simulink model "HvCoorn"  (R2022b)
settings: configuration reference "Icar05FusaMdlCfg" (kept outside this file)
undefined symbols (not defined in the file): BMSActSt_ACChrg, BMSActSt_DCChrg, BMSActSt_disconnect, BMSActSt_offline, BMSActSt_online, BMSActSt_undefined, BMSMainNegRlySt_Clsd_SC, BMSMainNegRlySt_Open_SC, BMSMainNegRlySt_StuckInClsd_SC, BMSMainNegRlySt_StuckInOpen_SC, BMSMainPosRlySt_Clsd_SC, BMSMainPosRlySt_Open_SC, BMSMainPosRlySt_StuckInClsd_SC, BMSPrecRlySt_StuckInOpen_SC, BMSReqSt_ACChrg, BMSReqSt_DCChrg, BMSReqSt_emergencyOffline, BMSReqSt_offline, BMSReqSt_online, Chrg_stCycleBookMod_SC, Chrg_stSingleBookMod_SC, CmpgMod_stInactv_SC, DCDCActSt_buck, DCDCActSt_connected, DCDCActSt_disconnected, DCDCReqSt_buck, DCDCReqSt_standby, EngStrtStop_RefuModDft_SC, EPBActSt_Appld_SC, GearLvr_stDrvGearD_SC, GearLvr_stDrvGearN_SC, GearLvr_stDrvGearP_SC, GearLvr_stDrvGearR_SC, hpp_bACChargeLinkIni_C, hpp_bACChargeLinkOKIni_C, hpp_bAcChgEnaIni_C, hpp_bAcChgPauseIni_C, hpp_bAcLinkTempErrIni_C, hpp_bBattWarmReqIni_C, hpp_bHvilHwErrIni_C, hpp_bHvilStOkIni_C, hpp_bHvRelayClsActIni_C, hpp_bHvRelayOpnActIni_C, hpp_bHvRelayStuckIni_C, hpp_bParked4ChDchgIni_C, hpp_bRemLvBatMntnReqIni_C, hpp_bStartUpReqIni_C, hpp_stHvilCanIni_C, hpp_stWarmTimeCfgRespIni_C, HvCoorn_bAuthEnaSwt_C, HvCoorn_bAuthFailSpdLimOvrd_C, HvCoorn_bAuthFailSpdLimOvrdVal_C, HvCoorn_bAuthStrt_C, HvCoorn_bBMSUnexpdDcnctFailEna_C, HvCoorn_bBuck2RdyBypDCDCEna_C, HvCoorn_bDCChrgFctCfg_C, HvCoorn_bDcChrgWkupEnaChrgLink_C, HvCoorn_bDCDcnct4ACEna_C, HvCoorn_bDCNotBuck2ShtdwnEna_C, HvCoorn_bDrvrLevNotRdyEna_C ... (+295)
libraries: ITKLib x213, simulink x61
(part 10 of 12)

== system HvCoorn/HvCoorn/HVP_HighVoltagePowerOnOffProcedure/A01_HighvoltPowerUpReq/B07_AcChrgPwrUp ==
  note: This subsystem calculates AC charge enable flag and AC charge wake up vehicle high voltage power up flag.
  note: Documentation
  HvCoorn_bACLinkTempErr : Inport
  HvCoorn_bParked4ChDchg : Inport  Port=2
  Chrg_bACChrgCmpl : Inport  Port=3
  iud_stOBCWakeUpOrigin : Inport  Port=4
  icobc_bChrgrCtrlSigCnct : Inport  Port=5
  icbms_bBatACChrgFull : Inport  Port=6
  Chrg_stBookChrgMod : Inport  Port=7
  HvCoorn_bObcChrgrCnct : Inport  Port=8
  HvCoorn_bACChrgLink : Inport  Port=9
  icobc_pwrChrgMax : Inport  Port=10
  HvCoorn_bBattWarmReq : Inport  Port=11
  Chrg_bBookChrgCmpl : Inport  Port=12
  HvCoorn_bACChrgLinkOk : Inport  Port=13
  Chrg_bChrgStopBySOCLim : Inport  Port=14
  Chrg_bChrgErrForever : Inport  Port=15
  Constant10 : Constant  Description=[254]  Value=HvCoorn_noACChrgEna_C
      settings: AttributesFormatString=%<Description>
  Copyright : simulink/Model-Wide Utilities/Model Info  Frame=on  DisplayStringWithTags=|  HorizontalTextAlignment=Left  LeftAlignmentValue=0.02
      | © ITK Engineering Technology (Wu Xi) Co., Ltd. (ITKC)
      | 
      | Model Version: %<ModelVersion>
      | Date: %<LastModificationDate>
  InlineDescription : ITKLib/Special/InlineDescription  Tag=HideFromReport  Description=AC充电上高压  ShowInLibBrowser=0  RefreshPar=0
      settings: SourceProductName=ITKC_Lib
  Logical Operator1 : Logic  AllPortsSameDT=off  OutDataTypeStr=boolean
  Logical Operator{2,4..5,10,24} (5 alike) : Logic  Operator=NOT  Inputs=1  AllPortsSameDT=off  OutDataTypeStr=boolean
  Logical Operator17 : Logic  Operator=OR  Inputs=3  AllPortsSameDT=off  OutDataTypeStr=boolean
  Logical Operator18 : Logic  AllPortsSameDT=off  OutDataTypeStr=boolean
  Logical Operator20 : Logic  Operator=OR  Inputs=3  AllPortsSameDT=off  OutDataTypeStr=boolean
  Logical Operator23 : Logic  Operator=OR  AllPortsSameDT=off  OutDataTypeStr=boolean
  Logical Operator31 : Logic  Operator=OR  AllPortsSameDT=off  OutDataTypeStr=boolean
  MaskAnd : ITKLib/BitOperation/MaskAnd
      settings: SourceProductName=ITKC_Lib
  Merge8bit2out : ITKLib/BitOperation/Merge8bit2out
      settings: AttributesFormatString=Merge8bit2out  SourceProductName=ITKC_Lib
  OR : Logic  Operator=OR  Inputs=3  OutDataTypeStr=boolean
  RSLatch : ITKLib/Memory/RSLatch
      settings: SourceProductName=ITKC_Lib
  RSLatch1 : ITKLib/Memory/RSLatch
      settings: SourceProductName=ITKC_Lib
  Relational Operator{3,5..6,10..11} (5 alike) : RelationalOperator  Operator===  OutDataTypeStr=boolean  InputSameDT=off
  Relational Operator7 : RelationalOperator  OutDataTypeStr=boolean  InputSameDT=off
  Unit Delay3 : UnitDelay  SampleTime=-1  HasFrameUpgradeWarning=on
      settings: AttributesFormatString=<initial=%<X0>>
  Unit detailed design : simulink/Model-Wide Utilities/DocBlock  Tag=HideFromReport  DocumentType=Text
      content=|
      | SMiVCU-3258 - AC充电使能
      | 以下条件同时满足，则激活[AC充电使能]：
      | 1.<充电激活输出状态>激活，且<OBC充电连接状态>为0x2：Connected激活并锁存，[AC充电连接标志位]为0时Reset；
      | 2.[AC充电连接OK标志位]为1且<BMS充电使能>为0x1：Enable；
      | 3.[停车运行充放电标志位]为1；
      | 4.<OBC当前可输出最大功率>大于一定值（HvCoorn_pwrOBCSplyLim_C，初始值500V）；
      | 5.<交流充电充满标志位>为0x0：Not full；
      | 6.<充电持续故障>为0；
      |
      | SMiVCU-3259 - AC充电高压请求标志位
      | [AC充电使能]激活且<AC充电完成标志位>为0在，则激活并锁存[AC充电高压请求标志位]，<AC充电完成标志位>为1Reset。
  hpp_bEpbPark4ChDchgEna_C4 : Constant  Description=[3]  Value=Chrg_stCycleBookMod_SC
      settings: AttributesFormatString=%<Description>
  hpp_bEpbPark4ChDchgEna_C5 : Constant  Description=[2]  Value=Chrg_stSingleBookMod_SC
      settings: AttributesFormatString=%<Description>
  hpp_pwrIpsSplyLim_C : Constant  Description=[0]  Value=HvCoorn_pwrOBCSplyLim_C
      settings: AttributesFormatString=%<Description>
  uint1 : Constant  Description=CCWake  Value=96  OutDataTypeStr=uint8
      settings: AttributesFormatString=|
      | %<OutDataTypeStr>
      | %<Description>
  uint2 : Constant  Description=CPWake  Value=97  OutDataTypeStr=uint8
      settings: AttributesFormatString=|
      | %<OutDataTypeStr>
      | %<Description>
  uint8 : Constant  Description=IgWake  Value=18  OutDataTypeStr=uint8
      settings: AttributesFormatString=|
      | %<OutDataTypeStr>
      | %<Description>
  HvCoorn_bACChrgEna : Outport  VectorParamsAs1DForOutWhenUnconnected=off
  HvCoorn_bACChrgPwrUp : Outport  Port=2  VectorParamsAs1DForOutWhenUnconnected=off
  wires:
  Logical Operator10/1 -> Logical Operator1/2
  Logical Operator1/1 -> RSLatch1/1
  iud_stOBCWakeUpOrigin/1 -> Relational Operator5/1, Relational Operator3/1, Relational Operator6/1
  uint2/1 -> Relational Operator6/2
  Relational Operator5/1 -> Logical Operator17/1
  Logical Operator18/1 -> Unit Delay3/1
  Logical Operator17/1 -> Logical Operator20/1  "WakeUpOrigin"
  Unit Delay3/1 -> Logical Operator20/2  "RePlugOrSwipCard"
  icbms_bBatACChrgFull/1 -> Logical Operator24/1
  Logical Operator24/1 -> Logical Operator23/1
  HvCoorn_bBattWarmReq/1 -> Logical Operator23/2
  Relational Operator6/1 -> Logical Operator17/3
  Relational Operator3/1 -> Logical Operator17/2
  uint1/1 -> Relational Operator3/2
  uint8/1 -> Relational Operator5/2
  MaskAnd/1 -> Logical Operator1/1, HvCoorn_bACChrgEna/1
  icobc_bChrgrCtrlSigCnct/1 -> Merge8bit2out/2, Logical Operator18/1
  HvCoorn_bObcChrgrCnct/1 -> Logical Operator18/2
  Chrg_stBookChrgMod/1 -> Relational Operator10/1, Relational Operator11/1
  hpp_bEpbPark4ChDchgEna_C4/1 -> Relational Operator10/2
  hpp_bEpbPark4ChDchgEna_C5/1 -> Relational Operator11/2
  Relational Operator11/1 -> Logical Operator31/2
  Relational Operator10/1 -> Logical Operator31/1
  Logical Operator31/1 -> Logical Operator20/3  "BookChg"
  RSLatch1/1 -> HvCoorn_bACChrgPwrUp/1  "HvCoorn_bACChrgPwrUp"
  Logical Operator20/1 -> RSLatch/1
  HvCoorn_bACChrgLink/1 -> Logical Operator2/1
  Logical Operator2/1 -> RSLatch/2
  RSLatch/1 -> Merge8bit2out/1  "bAcChgTrig"
  HvCoorn_bACLinkTempErr/1 -> Logical Operator5/1
  HvCoorn_bParked4ChDchg/1 -> Merge8bit2out/5
  Logical Operator5/1 -> Merge8bit2out/4
  Logical Operator23/1 -> Merge8bit2out/7
  Relational Operator7/1 -> Merge8bit2out/6
  hpp_pwrIpsSplyLim_C/1 -> Relational Operator7/2
  icobc_pwrChrgMax/1 -> Relational Operator7/1
  Chrg_bChrgErrForever/1 -> Logical Operator4/1
  Logical Operator4/1 -> Merge8bit2out/8
  Merge8bit2out/1 -> MaskAnd/1  "HvCoorn_noACChrgEnaBitVal"
  Constant10/1 -> MaskAnd/2
  HvCoorn_bACChrgLinkOk/1 -> Merge8bit2out/3
  OR/1 -> RSLatch1/2, Logical Operator10/1
  Chrg_bChrgStopBySOCLim/1 -> OR/2
  Chrg_bACChrgCmpl/1 -> OR/1
  Chrg_bBookChrgCmpl/1 -> OR/3

== system HvCoorn/HvCoorn/HVP_HighVoltagePowerOnOffProcedure/A01_HighvoltPowerUpReq/B08_DcChrgPwrUp ==
  note: This subsystem calculates DC charge enable flag and DC charge wake up vehicle high voltage power up flag.
  note: Documentation
  Chrg_bChrgStopBySOCLim : Inport
  Chrg_bChrgErrForever : Inport  Port=2
  HvCoorn_bDcLinkTempErr : Inport  Port=3
  HvCoorn_bParked4ChDchg : Inport  Port=4
  HvCoorn_bDCChrgLink : Inport  Port=5
  icbms_bDcChrgCfg : Inport  Port=6
  Chrg_bDCChrgCmpl : Inport  Port=7
  icbms_bBatDCChrgFull : Inport  Port=8
  icbms_uDcChgrCap : Inport  Port=9
  icbms_iDcChgrCap : Inport  Port=10
  icbms_bDcChrgWkup : Inport  Port=11
  AND : Logic  Inputs=8  OutDataTypeStr=boolean
  AND1 : Logic  OutDataTypeStr=boolean
  Copyright : simulink/Model-Wide Utilities/Model Info  Frame=on  DisplayStringWithTags=|  HorizontalTextAlignment=Left  LeftAlignmentValue=0.02
      | © ITK Engineering Technology (Wu Xi) Co., Ltd. (ITKC)
      | 
      | Model Version: %<ModelVersion>
      | Date: %<LastModificationDate>
  GreaterOrEqual : RelationalOperator  OutDataTypeStr=boolean
  InlineDescription : ITKLib/Special/InlineDescription  Tag=HideFromReport  Description=DC充电上高压  ShowInLibBrowser=0  RefreshPar=0
      settings: SourceProductName=ITKC_Lib
  Logical Operator1 : Logic  Operator=NOT  AllPortsSameDT=off  OutDataTypeStr=boolean
  Logical Operator2 : Logic  Operator=NOT  AllPortsSameDT=off  OutDataTypeStr=boolean
  Logical Operator4 : Logic  Operator=NOT  Inputs=1  AllPortsSameDT=off  OutDataTypeStr=boolean
  Logical Operator9 : Logic  Operator=NOT  AllPortsSameDT=off  OutDataTypeStr=boolean
  OR : Logic  Operator=OR  OutDataTypeStr=boolean
  Product : Product  InputSameDT=on  SaturateOnIntegerOverflow=on
  RSLatch : ITKLib/Memory/RSLatch
      settings: SourceProductName=ITKC_Lib
  Unit detailed design : simulink/Model-Wide Utilities/DocBlock  Tag=HideFromReport  DocumentType=Text
      content=|
      | SMiVCU-3265 - DC充电使能
      | 以下条件同时满足，则激活[DC充电使能]：
      | 1.[DC充电连接标志位]为1;
      | 2.[DC充电充满标志位]为0；
      | 3.[停车运行充放电标志位]为1；
      | 4.<直流充电激活状态>为1；
      | 5.<充电持续故障>为0；
      |
      | SMiVCU-3266 - DC充电高压请求标志位
      | [DC充电使能]激活，且<DC充电完成标志位>为0，则激活并锁存[DC充电高压请求标志位]，<DC充电完成标志位>为1则Reset。
  hpp_pwrIpsSplyLim_C1 : Constant  Description=[0]  Value=HvCoorn_pwrDCChrgrSplyLim_C
      settings: AttributesFormatString=%<Description>
  HvCoorn_bDCChrgEna : Outport  VectorParamsAs1DForOutWhenUnconnected=off
  HvCoorn_bDCChrgPwrUp : Outport  Port=2  VectorParamsAs1DForOutWhenUnconnected=off
  wires:
  AND/1 -> HvCoorn_bDCChrgEna/1, AND1/1
  Logical Operator2/1 -> AND1/2
  AND1/1 -> RSLatch/1
  RSLatch/1 -> HvCoorn_bDCChrgPwrUp/1  "HvCoorn_bDCChrgPwrUp"
  icbms_bBatDCChrgFull/1 -> Logical Operator9/1
  HvCoorn_bDCChrgLink/1 -> AND/1
  icbms_bDcChrgCfg/1 -> AND/2
  Logical Operator9/1 -> AND/3
  HvCoorn_bDcLinkTempErr/1 -> Logical Operator1/1
  Logical Operator1/1 -> AND/4
  HvCoorn_bParked4ChDchg/1 -> AND/5
  icbms_uDcChgrCap/1 -> Product/1
  icbms_iDcChgrCap/1 -> Product/2
  hpp_pwrIpsSplyLim_C1/1 -> GreaterOrEqual/2
  Product/1 -> GreaterOrEqual/1
  GreaterOrEqual/1 -> AND/6
  icbms_bDcChrgWkup/1 -> AND/7
  Chrg_bChrgErrForever/1 -> Logical Operator4/1
  Logical Operator4/1 -> AND/8
  OR/1 -> Logical Operator2/1, RSLatch/2
  Chrg_bDCChrgCmpl/1 -> OR/1
  Chrg_bChrgStopBySOCLim/1 -> OR/2

== system HvCoorn/HvCoorn/HVP_HighVoltagePowerOnOffProcedure/A01_HighvoltPowerUpReq/B09_KeyOnPwrUp ==
  note: Documentation
  idi_bKeyOn : Inport
  icbms_pctHVBatSOCDisp : Inport  Port=2
  PwrLimBatt_pwrMaxHvesDChrg : Inport  Port=3
  idi_bKeyStrt : Inport  Port=4
  HvCoorn_bHvReady : Inport  Port=5
  BrkPedDev_bBrk : Inport  Port=6
  iczcu_bHVPwrOffReq : Inport  Port=7
  HvCoorn_stHVPOld : Inport  Port=8
  icicm_bPwrOffReq : Inport  Port=9
  GearLvr_stDrvGear : Inport  Port=10
  HvCoorn_bChrgLink : Inport  Port=11
  icicm_bOTAOn : Inport  Port=12
  DrvMod_bVehShowMod : Inport  Port=13
  icbms_stHvBat : Inport  Port=14
  AND : Logic  OutDataTypeStr=boolean
  AND1 : Logic  Inputs=3  OutDataTypeStr=boolean
  Copyright : simulink/Model-Wide Utilities/Model Info  Frame=on  DisplayStringWithTags=|  HorizontalTextAlignment=Left  LeftAlignmentValue=0.02
      | © ITK Engineering Technology (Wu Xi) Co., Ltd. (ITKC)
      | 
      | Model Version: %<ModelVersion>
      | Date: %<LastModificationDate>
  EdgeFalling : ITKLib/Memory/EdgeFalling  Tag=initial value = 0
      settings: SourceProductName=ITKC_Lib
  EdgeRising : ITKLib/Memory/EdgeRising  Tag=initial value = 0
      settings: SourceProductName=ITKC_Lib
  EdgeRising1 : ITKLib/Memory/EdgeRising  Tag=initial value = 0
      settings: SourceProductName=ITKC_Lib
  EdgeRising2 : ITKLib/Memory/EdgeRising  Tag=initial value = 0
      settings: SourceProductName=ITKC_Lib
  Equal : RelationalOperator  Operator===  OutDataTypeStr=boolean  RndMeth=Simplest  InputSameDT=off
  Equal1 : RelationalOperator  Operator===  OutDataTypeStr=boolean  RndMeth=Simplest  InputSameDT=off
  HysteresisB : ITKLib/Hysteresis/HysteresisB  Description=HysteresisB
      settings: AttributesFormatString=%<Description>  SourceProductName=ITKC_Lib
  InlineDescription : ITKLib/Special/InlineDescription  Tag=HideFromReport  Description=KeyOn上高压  ShowInLibBrowser=0  RefreshPar=0
      settings: SourceProductName=ITKC_Lib
  Logical Operator{1,3..5,7} (5 alike) : Logic  AllPortsSameDT=off  OutDataTypeStr=boolean
  Logical Operator14 : Logic  Operator=NOT  Inputs=1  AllPortsSameDT=off  OutDataTypeStr=boolean
  Logical Operator15 : Logic  Inputs=3  AllPortsSameDT=off  OutDataTypeStr=boolean
  Logical Operator2 : Logic  Inputs=3  AllPortsSameDT=off  OutDataTypeStr=boolean
  LowerOrEqual : RelationalOperator  Operator=<=  OutDataTypeStr=boolean
  LowerOrEqual1 : RelationalOperator  OutDataTypeStr=boolean
  LowerOrEqual2 : RelationalOperator  Operator===  OutDataTypeStr=boolean
  NOT : Logic  Operator=NOT  AllPortsSameDT=off  OutDataTypeStr=boolean
  NOT1 : Logic  Operator=NOT  AllPortsSameDT=off  OutDataTypeStr=boolean
  Not : Logic  Operator=NOT  AllPortsSameDT=off  OutDataTypeStr=boolean
  Not1 : Logic  Operator=NOT  AllPortsSameDT=off  OutDataTypeStr=boolean
  Not2 : Logic  Operator=NOT  AllPortsSameDT=off  OutDataTypeStr=boolean
  OR{,1..2,4,6..7} (6 alike) : Logic  Operator=OR  OutDataTypeStr=boolean
  OR3 : Logic  OutDataTypeStr=boolean
  OR5 : Logic  Inputs=4  OutDataTypeStr=boolean
  OR8 : Logic  Operator=OR  Inputs=3  OutDataTypeStr=boolean
  RSLatch : ITKLib/Memory/RSLatch
      settings: SourceProductName=ITKC_Lib
  RSLatch1 : ITKLib/Memory/RSLatch
      settings: SourceProductName=ITKC_Lib
  Relational Operator3 : RelationalOperator  Operator=<  OutDataTypeStr=boolean  InputSameDT=off
  Relational Operator4 : RelationalOperator  Operator=<  OutDataTypeStr=boolean  InputSameDT=off
  Relational Operator5 : RelationalOperator  Operator=~=  OutDataTypeStr=boolean  InputSameDT=off
  Relational Operator6 : RelationalOperator  Operator=~=  OutDataTypeStr=boolean  InputSameDT=off
  Switch : Switch  Criteria=u2 ~= 0  SaturateOnIntegerOverflow=off  InputSameDT=off
      settings: AttributesFormatString=Criteria : %<Criteria>
  Switch1 : Switch  Criteria=u2 ~= 0  SaturateOnIntegerOverflow=off  InputSameDT=off
      settings: AttributesFormatString=Criteria : %<Criteria>
  TRUE : Constant  Description=TRUE  OutDataTypeStr=boolean
      settings: AttributesFormatString=%<Description>
  TRUE1 : Constant  Description=TRUE  OutDataTypeStr=boolean  SampleTime=-1
      settings: AttributesFormatString=%<Description>
  TaskTime_s1 : Constant  Value=TaskTime_10ms
      settings: AttributesFormatString=[0.01]
  TaskTime_s2 : Constant  Value=TaskTime_10ms
      settings: AttributesFormatString=[0.01]
  TaskTime_s3 : Constant  Value=TaskTime_10ms
      settings: AttributesFormatString=[0.01]
  TurnOnDelayVari1 : ITKLib/TimeCounter/TurnOnDelayVari
      settings: AttributesFormatString=TurnOnDelay  SourceProductName=ITKC_Lib
  TurnOnDelayVari2 : ITKLib/TimeCounter/TurnOnDelayVari
      settings: AttributesFormatString=TurnOnDelay  SourceProductName=ITKC_Lib
  Turn_Off_Delay_Vari : ITKLib/TimeCounter/Turn_Off_Delay_Vari
      settings: AttributesFormatString=TurnOffDelay  SourceProductName=ITKC_Lib
  Unit detailed design : simulink/Model-Wide Utilities/DocBlock  Tag=HideFromReport  DocumentType=Text
      content=|
      | SMiVCU-3273 - KeyOn高压请求标志位
      | 以下条件同时满足，则激活[KeyOn高压请求标志位]：
      | 1.<整车电源模式>为0x1：On，TurnOnDelay一定时间（HvCoorn_tiKeyOnDly_C，初始值0.05s）出现上升沿，则激活并锁存。
      | 若<高压下电指令>为1 TurnOnDelay一定时间（HvCoorn_tiPwrOffDly4RstKeyOn_C，初始值0.2s），或<整车电源模式>为0x0：off，或当前时刻<高压系统状态>在115~130之间出现上升沿Reset；
      | 2.<电池SOC>大于等于一定值（HvCoorn_pctBatSOCLim4Shut_C，初始值0.01）或<电池最大放电功率>大于等于一定值（hpp_pwrBatDChrgLim4Shut_C，初始值1000W）；
  UnitDelay : UnitDelay  SampleTime=-1  HasFrameUpgradeWarning=on
      settings: AttributesFormatString=<Initial=%<x0>>
  hpp_bEpbPark4ChDchgEna_C2 : Constant  Description=[6]  Value=GearLvr_stDrvGearP_SC  OutDataTypeStr=uint8
      settings: AttributesFormatString=%<Description>
  hpp_bEpbPark4ChDchgEna_C4 : Constant  Description=[4]  Value=GearLvr_stDrvGearN_SC  OutDataTypeStr=uint8
      settings: AttributesFormatString=%<Description>
  hpp_percBatDchgSocThre_C : Constant  Description=[0]  Value=HvCoorn_pctBatSOCLim4Shut_C
      settings: AttributesFormatString=%<Description>
  hpp_percBatDchgSocThre_C1 : Constant  Description=[1]  Value=HvCoorn_bKeyOnStrtHvEna_C
      settings: AttributesFormatString=%<Description>
  hpp_percBatDchgSocThre_C2 : Constant  Description=[1]  Value=HvCoorn_bKeyStrtStrtHvEna_C
      settings: AttributesFormatString=%<Description>
  hpp_percBatDchgSocThre_C3 : Constant  Description=[1]  Value=HvCoorn_bSOPVehKeyOnStrtHvEna_C
      settings: AttributesFormatString=%<Description>
  hpp_percBatDchgSocThre_C4 : Constant  Description=[10]  Value=HvCoorn_tiVehShowLoSocInhbOn_C
      settings: AttributesFormatString=%<Description>
  hpp_percBatDchgSocThre_C5 : Constant  Description=[0.2]  Value=HvCoorn_tiPwrOffDly4RstKeyOn_C
      settings: AttributesFormatString=%<Description>
  hpp_percBatDchgSocThre_C6 : Constant  Description=[0.03]  Value=HvCoorn_tiKeyOnRisKeep_C
      settings: AttributesFormatString=%<Description>
  hpp_percBatDchgSocThre_C7 : Constant  Description=[0]  Value=HvCoorn_bZCUPwrOffEna_C
      settings: AttributesFormatString=%<Description>
  hpp_pwrSocHiBatDchgThre_C : Constant  Description=[-5000]  Value=HvCoorn_pwrBatDChrgLim4Shut_C
      settings: AttributesFormatString=%<Description>
  hpp_pwrSocHiBatDchgThre_C1 : Constant  Description=[1]  Value=HvCoorn_bVehShowLoSocInhbKeyOnEna_C
      settings: AttributesFormatString=%<Description>
  hpp_pwrSocHiBatDchgThre_C2 : Constant  Description=[6]  Value=HvCoorn_pctVehShowLoSocInhbOnUppr_C
      settings: AttributesFormatString=%<Description>
  hpp_pwrSocHiBatDchgThre_C3 : Constant  Description=[4]  Value=HvCoorn_pctVehShowLoSocInhbOnLowr_C
      settings: AttributesFormatString=%<Description>
  icbms_acCharge : Constant  Description=[9]  Value=BMSActSt_ACChrg  OutDataTypeStr=uint8
      settings: AttributesFormatString=[9]
  icbms_dcCharge : Constant  Description=[8]  Value=BMSActSt_DCChrg  OutDataTypeStr=uint8
      settings: AttributesFormatString=[8]
  single : Constant  Value=101  OutDataTypeStr=uint8  SampleTime=-1
      settings: AttributesFormatString=%<OutDataTypeStr>
  single1 : Constant  Value=130  OutDataTypeStr=uint8  SampleTime=-1
      settings: AttributesFormatString=%<OutDataTypeStr>
  single2 : Constant  Value=89  OutDataTypeStr=uint8  SampleTime=-1
      settings: AttributesFormatString=%<OutDataTypeStr>
  sup_tiKeyStrt_C1 : Constant  Description=[0]  Value=HvCoorn_bKeyStrtBypBrkSwt_C
      settings: AttributesFormatString=%<Description>
  HvCoorn_bKeyOnPwrUp : Outport  VectorParamsAs1DForOutWhenUnconnected=off
  HvCoorn_bShowModSocLo : Outport  Port=2  VectorParamsAs1DForOutWhenUnconnected=off
  wires:
  idi_bKeyOn/1 -> Logical Operator1/1, [idi_bKeyOn]
  Logical Operator15/1 -> HvCoorn_bKeyOnPwrUp/1  "HvCoorn_bKeyOnPwrUp"
  PwrLimBatt_pwrMaxHvesDChrg/1 -> Relational Operator4/1
  icbms_pctHVBatSOCDisp/1 -> [icbms_pctHVBatSOCDisp], Relational Operator3/1
  hpp_percBatDchgSocThre_C/1 -> Relational Operator3/2
  hpp_pwrSocHiBatDchgThre_C/1 -> Relational Operator4/2
  Relational Operator4/1 -> Logical Operator7/2
  Relational Operator3/1 -> Logical Operator7/1
  Logical Operator7/1 -> Logical Operator14/1
  Logical Operator14/1 -> Logical Operator15/2
  hpp_percBatDchgSocThre_C1/1 -> Logical Operator1/2
  hpp_percBatDchgSocThre_C2/1 -> Logical Operator2/2
  idi_bKeyStrt/1 -> Logical Operator2/1
  RSLatch/1 -> Switch/3
  Logical Operator3/1 -> Logical Operator15/1
  HvCoorn_bHvReady/1 -> UnitDelay/1
  TRUE/1 -> Switch/1
  Switch/1 -> Logical Operator3/2
  sup_tiKeyStrt_C1/1 -> OR1/2
  BrkPedDev_bBrk/1 -> OR1/1
  OR1/1 -> Logical Operator2/3
  Logical Operator2/1 -> RSLatch/1
  NOT/1 -> RSLatch/2
  OR/1 -> Switch/2
  hpp_percBatDchgSocThre_C3/1 -> OR/1
  UnitDelay/1 -> OR/2
  Turn_Off_Delay_Vari/1 -> RSLatch1/1  "HvCoorn_bKeyOnRisSet"
  iczcu_bHVPwrOffReq/1 -> OR4/1
  TaskTime_s2/1 -> TurnOnDelayVari1/2
  hpp_percBatDchgSocThre_C5/1 -> TurnOnDelayVari1/3
  RSLatch1/1 -> Logical Operator3/1
  OR2/1 -> EdgeRising1/1
  TurnOnDelayVari1/1 -> OR2/1
  EdgeRising1/1 -> OR7/1
  HvCoorn_stHVPOld/1 -> [HvCoorn_stHVPOld], LowerOrEqual/1, LowerOrEqual1/1
  single/1 -> LowerOrEqual1/2
  single1/1 -> LowerOrEqual/2
  LowerOrEqual/1 -> OR3/1
  LowerOrEqual1/1 -> OR3/2
  OR3/1 -> OR2/2
  OR5/1 -> TurnOnDelayVari1/1
  icicm_bPwrOffReq/1 -> OR4/2
  OR4/1 -> OR5/1
  GearLvr_stDrvGear/1 -> Equal/1, Equal1/1
  hpp_bEpbPark4ChDchgEna_C2/1 -> Equal/2
  hpp_bEpbPark4ChDchgEna_C4/1 -> Equal1/2
  Equal/1 -> OR6/1
  Equal1/1 -> OR6/2
  OR6/1 -> OR5/4
  HvCoorn_bChrgLink/1 -> Not/1
  Not/1 -> OR5/3
  NOT1/1 -> OR7/2
  [idi_bKeyOn] -> NOT1/1
  [idi_bKeyOn] -> NOT/1
  TaskTime_s3/1 -> Turn_Off_Delay_Vari/2
  hpp_percBatDchgSocThre_C6/1 -> Turn_Off_Delay_Vari/3
  OR7/1 -> RSLatch1/2
  hpp_percBatDchgSocThre_C7/1 -> OR5/2
  Logical Operator1/1 -> Logical Operator4/1, Logical Operator5/1, EdgeRising/1
  EdgeFalling/1 -> Logical Operator4/2
  icicm_bOTAOn/1 -> EdgeFalling/1
  Logical Operator4/1 -> OR8/2
  EdgeRising/1 -> OR8/3
  Logical Operator5/1 -> OR8/1
  single2/1 -> LowerOrEqual2/2
  LowerOrEqual2/1 -> EdgeRising2/1
  EdgeRising2/1 -> Logical Operator5/2
  [HvCoorn_stHVPOld] -> LowerOrEqual2/1
  OR8/1 -> Turn_Off_Delay_Vari/1
  Switch1/1 -> Not2/1, Logical Operator15/3
  TRUE1/1 -> Switch1/3
  AND/1 -> Switch1/2
  DrvMod_bVehShowMod/1 -> AND/1
  hpp_pwrSocHiBatDchgThre_C1/1 -> AND/2
  [icbms_pctHVBatSOCDisp] -> HysteresisB/2
  hpp_pwrSocHiBatDchgThre_C2/1 -> HysteresisB/1
  icbms_acCharge/1 -> Relational Operator6/2
  icbms_dcCharge/1 -> Relational Operator5/2
  icbms_stHvBat/1 -> Relational Operator5/1, Relational Operator6/1
  Relational Operator5/1 -> AND1/2
  Relational Operator6/1 -> AND1/1
  hpp_percBatDchgSocThre_C4/1 -> TurnOnDelayVari2/3
  TaskTime_s1/1 -> TurnOnDelayVari2/2
  AND1/1 -> TurnOnDelayVari2/1
  Not1/1 -> Switch1/1
  TurnOnDelayVari2/1 -> Not1/1
  Not2/1 -> HvCoorn_bShowModSocLo/1
  HysteresisB/1 -> AND1/3
  hpp_pwrSocHiBatDchgThre_C3/1 -> HysteresisB/3

== system HvCoorn/HvCoorn/HVP_HighVoltagePowerOnOffProcedure/A01_HighvoltPowerUpReq/B10_RemotePwrUp ==
  note: This subsystem calculates Tbox remote wake up vehicle high voltage power up flag.
  ictel_stHvBatPrecdng : Inport
  tcj_bHvBatPrecdngFinish : Inport  Port=2
  iczcu_stRmtChrgReq : Inport  Port=3
  iud_stRemoteImmo : Inport  Port=4
  ipf_bBD1CAN0x41CVld : Inport  Port=5
  ictcp_stRmtHvReq : Inport  Port=6
  idi_bKeyOn : Inport  Port=7
  icbms_pctHVBatSOCDisp : Inport  Port=8
  Equal : RelationalOperator  Operator===  OutDataTypeStr=boolean  RndMeth=Simplest  InputSameDT=off
  Equal1 : RelationalOperator  Operator===  OutDataTypeStr=boolean  RndMeth=Simplest  InputSameDT=off
  Logical Operator1 : Logic  Operator=OR  AllPortsSameDT=off  OutDataTypeStr=boolean
  Logical Operator34 : Logic  Operator=OR  Inputs=3  AllPortsSameDT=off  OutDataTypeStr=boolean
  Logical Operator35 : Logic  AllPortsSameDT=off  OutDataTypeStr=boolean
  Logical Operator36 : Logic  Operator=OR  AllPortsSameDT=off  OutDataTypeStr=boolean
  Logical Operator9 : Logic  Operator=OR  Inputs=3  AllPortsSameDT=off  OutDataTypeStr=boolean
  Not : Logic  Operator=NOT  AllPortsSameDT=off  OutDataTypeStr=boolean
  OR : Logic  Operator=OR  Inputs=3  OutDataTypeStr=boolean
  RSLatch : ITKLib/Memory/RSLatch
      settings: SourceProductName=ITKC_Lib
  RSLatch1 : ITKLib/Memory/RSLatch
      settings: SourceProductName=ITKC_Lib
  RSLatch2 : ITKLib/Memory/RSLatch
      settings: SourceProductName=ITKC_Lib
  Relational Operator10 : RelationalOperator  Operator=<  OutDataTypeStr=boolean  InputSameDT=off
  Relational Operator{3..5,14..17} (7 alike) : RelationalOperator  Operator===  OutDataTypeStr=boolean  InputSameDT=off
  TaskTime_s1 : Constant  Value=TaskTime_10ms
      settings: AttributesFormatString=[0.01]
  TaskTime_s2 : Constant  Value=TaskTime_10ms
      settings: AttributesFormatString=[0.01]
  Terminator : Terminator
  TurnOnDelayVari : ITKLib/TimeCounter/TurnOnDelayVari
      settings: AttributesFormatString=TurnOnDelay  SourceProductName=ITKC_Lib
  TurnOnDelayVari1 : ITKLib/TimeCounter/TurnOnDelayVari
      settings: AttributesFormatString=TurnOnDelay  SourceProductName=ITKC_Lib
  hpp_bReMoteImmoEna_C : Constant  Description=[1]  Value=HvCoorn_bRemImobEna_C  OutDataTypeStr=boolean
      settings: AttributesFormatString=%<Description>
  hpp_tiRemHvBatPrecdngSet_C : Constant  Description=[0.01]  Value=HvCoorn_tiRemHvBatPreCdngSet_C
      settings: AttributesFormatString=%<Description>
  hpp_tiRemLvBatMntnSet_C : Constant  Description=[0.01]  Value=HvCoorn_tiRemLvBatMntnSet_C
      settings: AttributesFormatString=%<Description>
  sup_percSocAdj4HvOn_C : Constant  Description=[15]  Value=HvCoorn_pctSocRmtHvRstThd_C
      settings: AttributesFormatString=%<Description>
  uint1 : Constant  Description=Cycle  Value=2  OutDataTypeStr=uint8
      settings: AttributesFormatString=|
      | %<OutDataTypeStr>
      | %<Description>
  uint2 : Constant  Description=Single  Value=4  OutDataTypeStr=uint8
      settings: AttributesFormatString=|
      | %<OutDataTypeStr>
      | %<Description>
  uint3 : Constant  Description=Start  Value=6  OutDataTypeStr=uint8
      settings: AttributesFormatString=|
      | %<OutDataTypeStr>
      | %<Description>
  uint4 : Constant  Description=HV active  OutDataTypeStr=uint8
      settings: AttributesFormatString=|
      | %<OutDataTypeStr>
      | %<Description>
  uint5 : Constant  Description=HV not active  Value=2  OutDataTypeStr=uint8
      settings: AttributesFormatString=|
      | %<OutDataTypeStr>
      | %<Description>
  uint6 : Constant  Description=Released  Value=2  OutDataTypeStr=uint8
      settings: AttributesFormatString=|
      | %<OutDataTypeStr>
      | %<Description>
  uint7 : Constant  Description=Charge Req  OutDataTypeStr=uint8
      settings: AttributesFormatString=|
      | %<OutDataTypeStr>
      | %<Description>
  uint8 : Constant  Description=Charge Finished  Value=2  OutDataTypeStr=uint8
      settings: AttributesFormatString=|
      | %<OutDataTypeStr>
      | %<Description>
  uint9 : Constant  Description=Charge Req  Value=0  OutDataTypeStr=uint8
      settings: AttributesFormatString=|
      | %<OutDataTypeStr>
      | %<Description>
  HvCoorn_bRemPwrUp : Outport  VectorParamsAs1DForOutWhenUnconnected=off
  wires:
  TaskTime_s2/1 -> TurnOnDelayVari/2
  Logical Operator34/1 -> TurnOnDelayVari/1  "bHvBatPrecdng"
  tcj_bHvBatPrecdngFinish/1 -> RSLatch/2
  iczcu_stRmtChrgReq/1 -> Relational Operator3/1, Relational Operator5/1, Relational Operator4/1
  hpp_tiRemHvBatPrecdngSet_C/1 -> TurnOnDelayVari/3
  TurnOnDelayVari1/1 -> RSLatch1/1
  RSLatch/1 -> Logical Operator1/2
  uint1/1 -> Relational Operator14/2
  uint2/1 -> Relational Operator15/2
  uint3/1 -> Relational Operator16/2
  Relational Operator14/1 -> Logical Operator34/1
  Relational Operator15/1 -> Logical Operator34/2
  Relational Operator16/1 -> Logical Operator34/3
  ictel_stHvBatPrecdng/1 -> Relational Operator15/1, Relational Operator16/1, Relational Operator14/1
  uint6/1 -> Relational Operator17/2
  iud_stRemoteImmo/1 -> Relational Operator17/1
  Logical Operator35/1 -> TurnOnDelayVari1/1
  Logical Operator36/1 -> Logical Operator35/2
  Relational Operator17/1 -> Logical Operator36/1
  hpp_bReMoteImmoEna_C/1 -> Logical Operator36/2
  hpp_tiRemLvBatMntnSet_C/1 -> TurnOnDelayVari1/3
  Logical Operator1/1 -> HvCoorn_bRemPwrUp/1  "HvCoorn_bRemPwrUp"
  TurnOnDelayVari/1 -> RSLatch/1
  TaskTime_s1/1 -> TurnOnDelayVari1/2
  Relational Operator3/1 -> Logical Operator35/1
  uint7/1 -> Relational Operator3/2
  uint8/1 -> Relational Operator4/2
  Logical Operator9/1 -> RSLatch1/2
  uint9/1 -> Relational Operator5/2
  Relational Operator4/1 -> Logical Operator9/1
  Relational Operator5/1 -> Logical Operator9/2
  ipf_bBD1CAN0x41CVld/1 -> Not/1
  Not/1 -> Logical Operator9/3
  ictcp_stRmtHvReq/1 -> Equal1/1, Equal/1
  uint4/1 -> Equal/2
  Equal/1 -> RSLatch2/1
  RSLatch2/1 -> Logical Operator1/1
  Equal1/1 -> OR/1
  uint5/1 -> Equal1/2
  OR/1 -> RSLatch2/2
  idi_bKeyOn/1 -> OR/2
  RSLatch1/1 -> Terminator/1
  icbms_pctHVBatSOCDisp/1 -> Relational Operator10/1
  sup_percSocAdj4HvOn_C/1 -> Relational Operator10/2
  Relational Operator10/1 -> OR/3

== system HvCoorn/HvCoorn/HVP_HighVoltagePowerOnOffProcedure/A01_HighvoltPowerUpReq/B11_ECCPwrUp ==
  note: Documentation
  icecc_bHVReq : Inport
  icems_bFanAftRunActv : Inport  Port=2
  HvCoorn_bKeyOnPwrUp : Inport  Port=3
  AND : Logic  OutDataTypeStr=boolean
  AND1 : Logic  OutDataTypeStr=boolean
  Copyright : simulink/Model-Wide Utilities/Model Info  Frame=on  DisplayStringWithTags=|  HorizontalTextAlignment=Left  LeftAlignmentValue=0.02
      | © ITK Engineering Technology (Wu Xi) Co., Ltd. (ITKC)
      | 
      | Model Version: %<ModelVersion>
      | Date: %<LastModificationDate>
  EdgeFalling : ITKLib/Memory/EdgeFalling  Tag=initial value = 0
      settings: SourceProductName=ITKC_Lib
  InlineDescription : ITKLib/Special/InlineDescription  Tag=HideFromReport  Description=热管理上高压  ShowInLibBrowser=0  RefreshPar=0
      settings: SourceProductName=ITKC_Lib
  NormShut1 : Constant  Description=[1]  Value=HvCoorn_bECCPwrUpEna_C
      settings: AttributesFormatString=%<Description>
  Not : Logic  Operator=NOT  AllPortsSameDT=off  OutDataTypeStr=boolean
  OR : Logic  Operator=OR  OutDataTypeStr=boolean
  OR1 : Logic  Operator=OR  OutDataTypeStr=boolean
  RSLatch : ITKLib/Memory/RSLatch
      settings: SourceProductName=ITKC_Lib
  TaskTime_s1 : Constant  Value=TaskTime_10ms
      settings: AttributesFormatString=[0.01]
  TurnOnDelayVari1 : ITKLib/TimeCounter/TurnOnDelayVari
      settings: AttributesFormatString=TurnOnDelay  SourceProductName=ITKC_Lib
  Unit Delay : UnitDelay  SampleTime=-1  HasFrameUpgradeWarning=on
      settings: AttributesFormatString=<initial=%<x0>>
  Unit detailed design : simulink/Model-Wide Utilities/DocBlock  Tag=HideFromReport  DocumentType=Text
      content=|
      | SMiVCU-3269 - 热管理高压请求标志位
      | 以下条件同时满足，则激活[热管理高压请求标志位]：
      | 1.[热管理高压请求]为1；
      | 2.[热管理可用最大功率]大于一定值（HvCoorn_pwrEccEnaHv_C，初始值1W）。
  hpp_tiRemLvBatMntnSet_C : Constant  Description=[600]  Value=HvCoorn_tiFanAftRunMaxThd_C
      settings: AttributesFormatString=%<Description>
  HvCoorn_bECCPwrUp : Outport
  wires:
  icecc_bHVReq/1 -> AND/1
  NormShut1/1 -> AND/2
  HvCoorn_bKeyOnPwrUp/1 -> EdgeFalling/1
  EdgeFalling/1 -> AND1/1
  icems_bFanAftRunActv/1 -> Not/1, AND1/2
  AND/1 -> OR/1
  OR/1 -> HvCoorn_bECCPwrUp/1
  RSLatch/1 -> OR/2, Unit Delay/1  "HvCoorn_bFanAftRunPwrUp"
  AND1/1 -> RSLatch/1
  Not/1 -> OR1/1
  OR1/1 -> RSLatch/2
  hpp_tiRemLvBatMntnSet_C/1 -> TurnOnDelayVari1/3
  TaskTime_s1/1 -> TurnOnDelayVari1/2
  TurnOnDelayVari1/1 -> OR1/2
  Unit Delay/1 -> TurnOnDelayVari1/1

== system HvCoorn/HvCoorn/HVP_HighVoltagePowerOnOffProcedure/A01_HighvoltPowerUpReq/B12_OTAPwrUp ==
  icicm_bOTAOn : Inport
  icicm_stHVReq : Inport  Port=2
  AND : Logic  OutDataTypeStr=boolean
  AND1 : Logic  OutDataTypeStr=boolean
  Equal : RelationalOperator  Operator===  OutDataTypeStr=boolean  RndMeth=Simplest  InputSameDT=off
  Equal1 : RelationalOperator  Operator===  OutDataTypeStr=boolean  RndMeth=Simplest  InputSameDT=off
  uint1 : Constant  Value=2  OutDataTypeStr=uint8  SampleTime=-1
      settings: AttributesFormatString=%<OutDataTypeStr>
  uint8 : Constant  OutDataTypeStr=uint8  SampleTime=-1
      settings: AttributesFormatString=%<OutDataTypeStr>
  HvCoorn_bOTAPwrUp : Outport
  HvCoorn_bOTAHvOffReq : Outport  Port=2
  wires:
  icicm_stHVReq/1 -> Equal1/1, Equal/1
  uint8/1 -> Equal/2
  Equal/1 -> AND/2
  AND/1 -> HvCoorn_bOTAPwrUp/1
  icicm_bOTAOn/1 -> AND1/1, AND/1
  Equal1/1 -> AND1/2
  uint1/1 -> Equal1/2
  AND1/1 -> HvCoorn_bOTAHvOffReq/1

== system HvCoorn/HvCoorn/HVP_HighVoltagePowerOnOffProcedure/A01_HighvoltPowerUpReq/B13_GatherPwrUpReq ==
  note: This subsystem calculates high voltage start up request flag, based on AC charge, DC charge, Key on, remote power up.
  note: Documentation
  HvCoorn_bACChrgPwrUp : Inport
  HvCoorn_bDCChrgPwrUp : Inport  Port=2
  HvCoorn_bKeyOnPwrUp : Inport  Port=3
  ved_bHvShtdwn : Inport  Port=4
  icbms_bHvShutOffReq : Inport  Port=5
  HvCoorn_bRemPwrUp : Inport  Port=6
  HvCoorn_bECCPwrUp : Inport  Port=7
  HvCoorn_bOTAPwrUp : Inport  Port=8
  HvCoorn_bOTAHvOffReq : Inport  Port=9
  GearLvr_stDrvGear : Inport  Port=10
  icbms_pctHVBatSOCDisp : Inport  Port=11
  iczcu_stCarMod : Inport  Port=12
  HvCoorn_bV2LActv : Inport  Port=13
  ved_bInhbHvOn : Inport  Port=14
  HvCoorn_stHVPOld : Inport  Port=15
  HvCoorn_bHvOnFai : Inport  Port=16
  HvCoorn_bHvInitFail : Inport  Port=17
  HvCoorn_bRemLvBatMntnReq : Inport  Port=18
  RngPrdn_volFuRmnByInstModEEW : Inport  Port=19
  ved_bInhbEngStrt : Inport  Port=20
  ved_bCellVoltUndLimSrus : Inport  Port=21
  AND : Logic  Inputs=4  OutDataTypeStr=boolean
  AND1 : Logic  OutDataTypeStr=boolean
  AND2 : Logic  OutDataTypeStr=boolean
  Calibration6 : Constant  Description=[3]  Value=HvCoorn_volTankRmnFuLowrTranMod_C  SampleTime=-1
      settings: AttributesFormatString=%<Description>
  Copyright : simulink/Model-Wide Utilities/Model Info  Frame=on  DisplayStringWithTags=|  HorizontalTextAlignment=Left  LeftAlignmentValue=0.02
      | © ITK Engineering Technology (Wu Xi) Co., Ltd. (ITKC)
      | 
      | Model Version: %<ModelVersion>
      | Date: %<LastModificationDate>
  Equal1 : RelationalOperator  Operator=<=  OutDataTypeStr=boolean  RndMeth=Simplest  InputSameDT=off
  Equal2 : RelationalOperator  Operator===  OutDataTypeStr=boolean
  Equal3 : RelationalOperator  OutDataTypeStr=boolean  RndMeth=Simplest  InputSameDT=off
  Equal4 : RelationalOperator  Operator=<  OutDataTypeStr=boolean
  Equal5 : RelationalOperator  Operator===  OutDataTypeStr=boolean  RndMeth=Simplest  InputSameDT=off
  Equal6 : RelationalOperator  Operator===  OutDataTypeStr=boolean  RndMeth=Simplest  InputSameDT=off
  InlineDescription : ITKLib/Special/InlineDescription  Tag=HideFromReport  Description=高压上电请求  ShowInLibBrowser=0  RefreshPar=0
      settings: SourceProductName=ITKC_Lib
  Logical Operator{1..5} (5 alike) : Logic  Operator=NOT  Inputs=1  AllPortsSameDT=off  OutDataTypeStr=boolean
  Logical Operator26 : Logic  Inputs=6  AllPortsSameDT=off  OutDataTypeStr=boolean
  Merge8bit2out : ITKLib/BitOperation/Merge8bit2out
      settings: AttributesFormatString=Merge8bit2out  SourceProductName=ITKC_Lib
  Not : Logic  Operator=NOT  AllPortsSameDT=off  OutDataTypeStr=boolean
  OR : Logic  Operator=OR  Inputs=3  OutDataTypeStr=boolean
  OR1 : Logic  Operator=OR  Inputs=6  OutDataTypeStr=boolean
  OR2 : Logic  Operator=OR  OutDataTypeStr=boolean
  OR3 : Logic  Operator=OR  Inputs=3  OutDataTypeStr=boolean
  OR4 : Logic  Operator=OR  OutDataTypeStr=boolean
  OR5 : Logic  Operator=OR  OutDataTypeStr=boolean
  Relational Operator10 : RelationalOperator  Operator=<=  OutDataTypeStr=boolean  InputSameDT=off
  TaskTime_s1 : Constant  Description=[4]  Value=GearLvr_stDrvGearN_SC  SampleTime=-1
      settings: AttributesFormatString=%<Description>
  TaskTime_s2 : Constant  Description=[6]  Value=GearLvr_stDrvGearP_SC  SampleTime=-1
      settings: AttributesFormatString=%<Description>
  TaskTime_s3 : Constant  Value=TaskTime_10ms
      settings: AttributesFormatString=[0.01]
  TurnOnDelayVari : ITKLib/TimeCounter/TurnOnDelayVari
      settings: AttributesFormatString=TurnOnDelay  SourceProductName=ITKC_Lib
  Unit detailed design : simulink/Model-Wide Utilities/DocBlock  Tag=HideFromReport  DocumentType=Text
      content=|
      | SMiVCU-3271 - 上高压需求标志位
      | 以下任一条件满足，且<整车故障等级>小于4，且<BMS高压断开请求>为0，则激活[上高压需求标志位]
      | 1.[AC充电高压请求标志位]为1；
      | 2.[DC充电高压请求标志位]；
      | 3.[KeyOn高压请求标志位]；
      | 4.[热管理高压请求标志位]，且热管理上高压使能标志位（HvCoorn_bECCPwrUpEna_C，初始值0）为1。
  hpp_percBatDchgSocThre_C6 : Constant  Description=[0.3]  Value=HvCoorn_tiCarModPwrOffDly_C
      settings: AttributesFormatString=%<Description>
  sup_percSocAdj4HvOn_C : Constant  Description=[10]  Value=HvCoorn_pctSocTransptHvOff_C
      settings: AttributesFormatString=%<Description>
  uint1 : Constant  Value=2  OutDataTypeStr=uint8  SampleTime=-1
      settings: AttributesFormatString=%<OutDataTypeStr>
  uint2 : Constant  Value=10  OutDataTypeStr=uint8  SampleTime=-1
      settings: AttributesFormatString=%<OutDataTypeStr>
  uint3 : Constant  Value=101  OutDataTypeStr=uint8  SampleTime=-1
      settings: AttributesFormatString=%<OutDataTypeStr>
  HvCoorn_bStartUpReq : Outport  VectorParamsAs1DForOutWhenUnconnected=off
  HvCoorn_stStartUpReq : Outport  Port=2  VectorParamsAs1DForOutWhenUnconnected=off
  wires:
  HvCoorn_bACChrgPwrUp/1 -> OR/1, Merge8bit2out/1
  Logical Operator26/1 -> HvCoorn_bStartUpReq/1
  HvCoorn_bKeyOnPwrUp/1 -> Merge8bit2out/4, OR1/2
  HvCoorn_bRemPwrUp/1 -> OR1/1, Merge8bit2out/3
  HvCoorn_bDCChrgPwrUp/1 -> OR/2, Merge8bit2out/2
  Logical Operator1/1 -> Logical Operator26/2
  icbms_bHvShutOffReq/1 -> Logical Operator1/1
  HvCoorn_bECCPwrUp/1 -> OR1/4, Merge8bit2out/6
  Logical Operator2/1 -> Logical Operator26/3
  HvCoorn_bOTAPwrUp/1 -> Merge8bit2out/5, OR1/3
  HvCoorn_bOTAHvOffReq/1 -> Logical Operator3/1
  Logical Operator3/1 -> Logical Operator26/4
  Merge8bit2out/1 -> HvCoorn_stStartUpReq/1
  HvCoorn_bV2LActv/1 -> OR1/5, Merge8bit2out/7
  GearLvr_stDrvGear/1 -> Equal6/1, Equal5/1
  TaskTime_s2/1 -> Equal5/2
  sup_percSocAdj4HvOn_C/1 -> Relational Operator10/2
  icbms_pctHVBatSOCDisp/1 -> Relational Operator10/1
  uint1/1 -> Equal2/2  "TransportMode"
  iczcu_stCarMod/1 -> Equal2/1
  Relational Operator10/1 -> AND/2
  Equal2/1 -> AND/3
  AND/1 -> Not/1
  OR1/1 -> AND1/1
  AND1/1 -> OR/3
  OR/1 -> Logical Operator26/1
  ved_bHvShtdwn/1 -> Logical Operator2/1
  ved_bInhbHvOn/1 -> OR3/1
  AND2/1 -> Logical Operator4/1
  Logical Operator4/1 -> Logical Operator26/6
  HvCoorn_stHVPOld/1 -> Equal3/1, Equal1/1
  Equal1/1 -> OR2/1
  OR2/1 -> AND2/2
  Equal3/1 -> OR2/2
  uint2/1 -> Equal1/2
  uint3/1 -> Equal3/2
  OR3/1 -> AND2/1
  HvCoorn_bHvOnFai/1 -> OR3/2
  HvCoorn_bHvInitFail/1 -> OR3/3
  TaskTime_s3/1 -> TurnOnDelayVari/2
  hpp_percBatDchgSocThre_C6/1 -> TurnOnDelayVari/3
  Not/1 -> TurnOnDelayVari/1
  TurnOnDelayVari/1 -> AND1/2
  HvCoorn_bRemLvBatMntnReq/1 -> OR1/6, Merge8bit2out/8
  RngPrdn_volFuRmnByInstModEEW/1 -> Equal4/1
  Calibration6/1 -> Equal4/2
  Equal5/1 -> OR4/1
  OR4/1 -> AND/1
  Equal6/1 -> OR4/2
  TaskTime_s1/1 -> Equal6/2
  ved_bInhbEngStrt/1 -> OR5/2
  Equal4/1 -> OR5/1
  OR5/1 -> AND/4
  Logical Operator5/1 -> Logical Operator26/5
  ved_bCellVoltUndLimSrus/1 -> Logical Operator5/1
